simulink model "RECEIVER"  (R2024b)
settings: Solver=VariableStepAuto  StartTime=0.0  StopTime=inf  RelTol=1e-3
libraries: commsdrhw_v2 x1
settings Model: SimulationMode=accelerator  Creator=aravj  LastModifiedBy=aravj

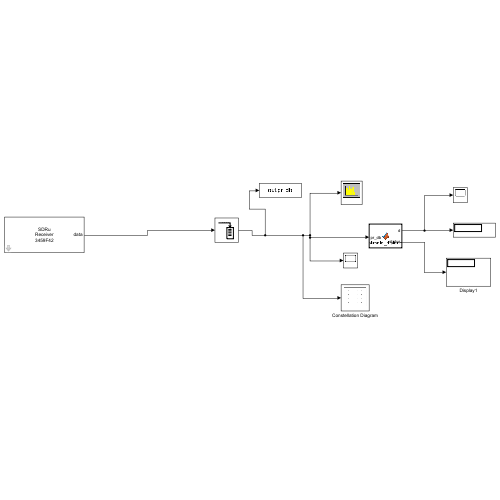
[thumbnail: Simulink's stored preview of the top-level diagram]
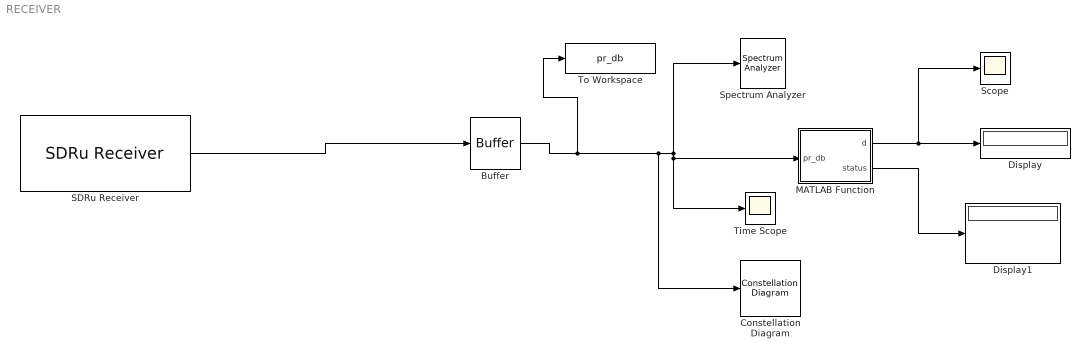
== system RECEIVER ==
  Buffer : Buffer  OutputFrames=off
  Constellation Diagram : ConstellationDiagram  DefaultConfigurationName=comm.scopes.ConstellationDiagramBlockCfg
  Display : Display
  Display1 : Display
  MATLAB Function : MATLAB Function  TreatAsAtomicUnit=on
  SDRu Receiver : commsdrhw_v2/SDRu Receiver  rxtx=rx  initializeIPAddress=0  devMap=10  USRP2_IP=192.168.10.2  USRP_IP_X300=192.168.10.2  USRP_IP_X310=No devices found  USRP_IP_N300=192.168.10.2  USRP_IP_N310=192.168.10.2  USRP_IP_N320=192.168.10.2  USRP_serialNumB200=3136D21  USRP_serialNumB210=3459F42  platform=B210  prevPlatform=B210  lastIPAddressPopup=192.168.10.2  USRP_ID=3459F42  LastIPAddress=192.168.10.2  IsTwinRXDaughterboard=off  EnableTwinRXPhaseSync=off  losrc=0  ChannelMapping=1  centerFrequencySrc=Dialog  centerFrequency=2.45e9  loOffsetSrc=Dialog  loOffset=0  gainSrc=Dialog  gain=25  PPSSource=Internal  clockSource=Internal  EnableGPSLock=off  EnsureSyncGPSTime=off  EnableTimeTrigger=off  triggerTime=5  enableMIMOCableSync=off  EnableRefLock=off  masterClkRateParam=10000000  masterClkRateB200=32e6  masterClkRateB210=10e6  masterClkRateX300=200e6  masterClkRateX310=200e6  masterClkRateN300=125e6  masterClkRateN310=125e6  masterClkRateN320=200e6  masterClkRate=100e6  masterClkRateTwinRX=200e6  decimInterpSrc=Dialog  decimInterpPort=512  lastDecimSource=Dialog  decimInterp=5  USRP2_IP_NUM=[51 52 53 57 70 52 50]  sampleRate=2000000  sampleTime=(5)/10000000  TransportDataType=int16  overrunUnderrunPort=off  dataLengthPort=off  EnableTimeStamps=off  outputDatatype=Same as transport data type  frameLength=2048  HOST_DATA_PORT=0  HOST_CONTROL_PORT=0  USRP2_DATA_PORT=0  USRP2_CONTROL_PORT=0  bufferMode=Continuous streaming  EnableBurstMode=off  NumFramesInBurst=100
  Scope : Scope
  Spectrum Analyzer : SpectrumAnalyzer  WindowPosition=[0.000000,36.000000,1536.000000,792.000000,]  ScopeFrameLocation=window  SampleRate=44.1e3  PlotAsTwoSidedSpectrum=off  FrequencyScale=Log  WindowInvariantSamplesPerUpdate=on  FrequencySpan=Start and stop frequencies  StartFrequency=20  StopFrequency=20e3  YLimits=[2.2656,61.318]  SelectedToolstripTab=spectrumAnalyzerToolstrip.measurementsTab
  Time Scope : Scope
  To Workspace : ToWorkspace  VariableName=pr_db  SampleTime=-1
  wires:
  Buffer/1 -> To Workspace/1, Constellation Diagram/1, MATLAB Function/1(pr_db), Time Scope/1, Spectrum Analyzer/1
  SDRu Receiver/1 -> Buffer/1
  MATLAB Function/1(d) -> Display/1, Scope/1
  MATLAB Function/2(status) -> Display1/1

== matlab function RECEIVER/MATLAB Function ==
  data: pr_db input; d output; status output
function [d,status] = estimate_distance(pr_db)
pr_db=double(pr_db);
pr_db=abs(pr_db).^2;
Pr = 10*log10(mean(pr_db(end-50:end)));   % average RSS

Pt = -10;   % dB
n  = 2.5;
C  = 0;

d = 10.^((Pt - Pr - C)/(10*n));
d = d*1200;
if d<20
    status="STOP";
else
    status="SAFE TO TRAVEL";
end
fprintf('Estimated distance = %.2f cm %s \n', d,status);
end
